simulink library "feedback_robot"  (R2018a)
settings: Solver=VariableStepAuto  StartTime=0.0  StopTime=10.0  RelTol=1e-3
undefined symbols (not defined in the file or in its folder): DiscIntNeverNeededParam, lowerLimit, upperLimit
libraries: simulink x1
settings Model: Creator=daniel  LastModifiedBy=daniel

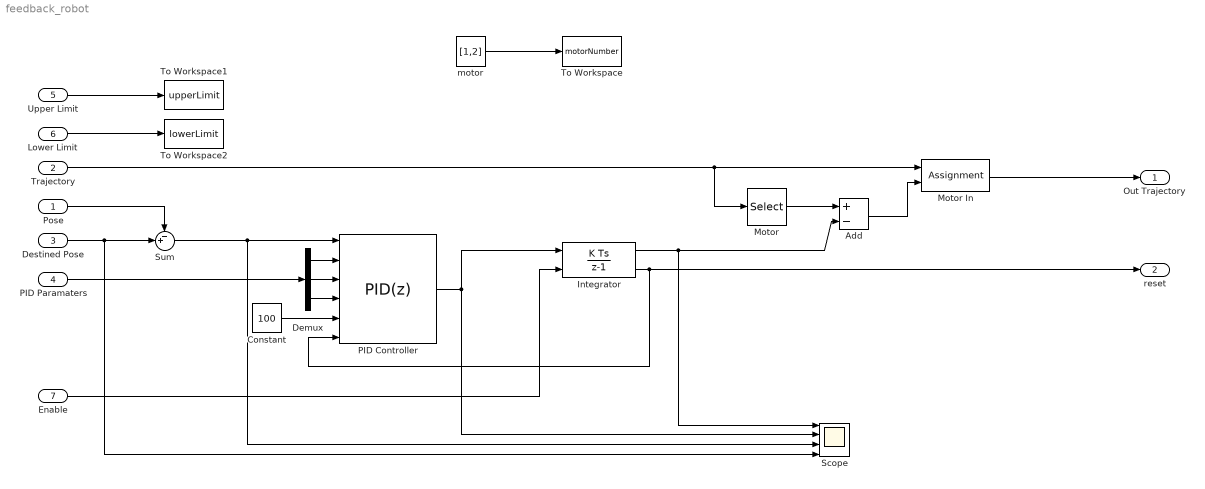
== system feedback_robot ==
  Pose : Inport
  Trajectory : Inport  Port=2
  Destined Pose : Inport  Port=3  OutDataTypeStr=single
  PID Paramaters : Inport  Port=4
  Upper Limit : Inport  Port=5
  Lower Limit : Inport  Port=6
  Enable : Inport  Port=7
  Add : Sum  Inputs=+-
  Constant : Constant  Value=100
  Demux : Demux  Outputs=3
  Integrator : DiscreteIntegrator  gainval=hipGain  ExternalReset=level  SampleTime=-1  LimitOutput=on  UpperSaturationLimit=upperLimit  LowerSaturationLimit=lowerLimit  ShowSaturationPort=on  ICPrevOutput=DiscIntNeverNeededParam  ICPrevScaledInput=DiscIntNeverNeededParam
  Motor : Selector  InputPortWidth=20  IndexOptions=Index vector (dialog)  Indices=motorNumber  OutputSizes=1
  Motor In : Assignment  DiagnosticForDimensions=Warning  IndexOptions=Index vector (dialog)  Indices=motorNumber  OutputSizes=1
  PID Controller : simulink/Continuous/PID Controller  Controller=PID  TimeDomain=Discrete-time  SampleTime=-1  IntegratorMethod=Forward Euler  FilterMethod=Forward Euler  Form=Parallel  UseFilter=on  ControllerParametersSource=external  P=0.5  I=1  D=0.001  N=100  InitialConditionSource=internal  InitialConditionForIntegrator=0  InitialConditionForFilter=0  ExternalReset=level  LimitOutput=off  UpperSaturationLimit=inf  LowerSaturationLimit=-inf  LinearizeAsGain=on  AntiWindupMode=none  Kb=1  TrackingMode=off  Kt=1  PParamMin=[]  PParamMax=[]  IParamMin=[]  IParamMax=[]  DParamMin=[]  DParamMax=[]  NParamMin=[]  NParamMax=[]  KbParamMin=[]  KbParamMax=[]  KtParamMin=[]  KtParamMax=[]  POutMin=[]  POutMax=[]  IOutMin=[]  IOutMax=[]  DOutMin=[]  DOutMax=[]  NOutMin=[]  NOutMax=[]  KbOutMin=[]  KbOutMax=[]  KtOutMin=[]  KtOutMax=[]  IntegratorOutMin=[]  IntegratorOutMax=[]  FilterOutMin=[]  FilterOutMax=[]  SumOutMin=[]  SumOutMax=[]  SumI1OutMin=[]  SumI1OutMax=[]  SumI2OutMin=[]  SumI2OutMax=[]  SumI3OutMin=[]  SumI3OutMax=[]  SumDOutMin=[]  SumDOutMax=[]  SaturationOutMin=[]  SaturationOutMax=[]  IntegratorContinuousStateAttributes=''  IntegratorStateMustResolveToSignalObject=off  IntegratorRTWStateStorageClass=Auto  FilterContinuousStateAttributes=''  FilterStateMustResolveToSignalObject=off  FilterRTWStateStorageClass=Auto  DifferentiatorICPrevScaledInput=0  DifferentiatorOutMin=[]  DifferentiatorOutMax=[]  FilterDiffOutCoefMin=[]  FilterDiffOutCoefMax=[]  SumDenOutMin=[]  SumDenOutMax=[]  SumNumOutMin=[]  SumNumOutMax=[]  ReciprocalOutMin=[]  ReciprocalOutMax=[]  DivideOutMin=[]  DivideOutMax=[]  TunerSelectOption=Transfer Function Based (PID Tuner App)
  Scope : Scope  NumInputPorts=4
  Sum : Sum  Inputs=-+|
  To Workspace : ToWorkspace  VariableName=motorNumber  SaveFormat=Timeseries  SampleTime=-1
  To Workspace1 : ToWorkspace  VariableName=upperLimit  SaveFormat=Timeseries  SampleTime=-1
  To Workspace2 : ToWorkspace  VariableName=lowerLimit  SaveFormat=Timeseries  SampleTime=-1
  motor : Constant  Value=[1,2]
  Out Trajectory : Outport
  reset : Outport  Port=2
  wires:
  Add/1 -> Motor In/2
  Sum/1 -> Scope/3, PID Controller/1
  Motor/1 -> Add/1
  Trajectory/1 -> Motor In/1, Motor/1
  Enable/1 -> Integrator/2
  motor/1 -> To Workspace/1
  Motor In/1 -> Out Trajectory/1
  Destined Pose/1 -> Sum/2, Scope/4
  PID Controller/1 -> Integrator/1, Scope/2
  Demux/1 -> PID Controller/2
  Demux/2 -> PID Controller/3
  Demux/3 -> PID Controller/4
  PID Paramaters/1 -> Demux/1
  Integrator/1 -> Add/2, Scope/1
  Upper Limit/1 -> To Workspace1/1
  Lower Limit/1 -> To Workspace2/1
  Constant/1 -> PID Controller/5
  Pose/1 -> Sum/1
  Integrator/2 -> PID Controller/6, reset/1
